simulink model "model_Q2"  (R2023b)
settings: Solver=ode45  StartTime=0.0  StopTime=25  RelTol=1e-5  AbsTol=1e-5  EnableMultiTasking=on
undefined symbols (not defined in the file or in its folder): control_Q2, vr
settings Model: Creator=pmorin  LastModifiedBy=baovi
settings SolverCC: AutoScaleAbsTol=off  AlgebraicLoopSolver=TrustRegion
settings DataIOCC: LimitDataPoints=on  SaveFormat=Array  SignalLoggingSaveFormat=ModelDataLogs  ReturnWorkspaceOutputs=off
settings OptimizationCC: BooleanDataType=off  ExpressionDepthLimit=2147483647  LifeSpan=inf
settings DebuggingCC: SaveWithParameterizedLinksMsg=none  UnderspecifiedInitializationDetection=Classic  MergeDetectMultiDrivingBlocksExec=none  SignalResolutionControl=TryResolveAllWithWarning  MultiTaskDSMMsg=warning  MultiTaskCondExecSysMsg=none  FcnCallInpInsideContextMsg=warning  UnconnectedInputMsg=warning  UnconnectedOutputMsg=warning  UnconnectedLineMsg=warning  StateNameClashWarn=warning  SFUnexpectedBacktrackingDiag=warning  SFNoUnconditionalDefaultTransitionDiag=warning  SFExecutionAtInitializationDiag=none  ArithmeticOperatorsInVariantConditions=warning
settings HardwareCC: ProdBitPerPointer=32  ProdBitPerSizeT=32  ProdBitPerPtrDiffT=32  ProdLargestAtomicFloat=None  ProdIntDivRoundTo=Undefined  ProdEndianess=Unspecified  ProdWordSize=32  ProdHWDeviceType=32-bit Generic  TargetUnknown=on
settings ModelReferenceCC: EnableRefExpFcnMdlSchedulingChecks=on  PropagateSignalLabelsOutOfModel=off
settings SFSimCC: SimUseLocalCustomCode=off  CustomCodeUndefinedFunction=UseInterfaceOnly
settings RTWCC: RTWUseLocalCustomCode=off
settings CodeAppCC: StateflowObjectComments=on
settings GRTTargetCC: TargetLangStandard=C89/C90 (ANSI)  CombineOutputUpdateFcns=off  GRTInterface=on
settings ConfigComp: CovMetricSettings=dw  CovSaveCumulativeToWorkspaceVar=on  CovSaveSingleToWorkspaceVar=on  CovExternalEMLEnable=off

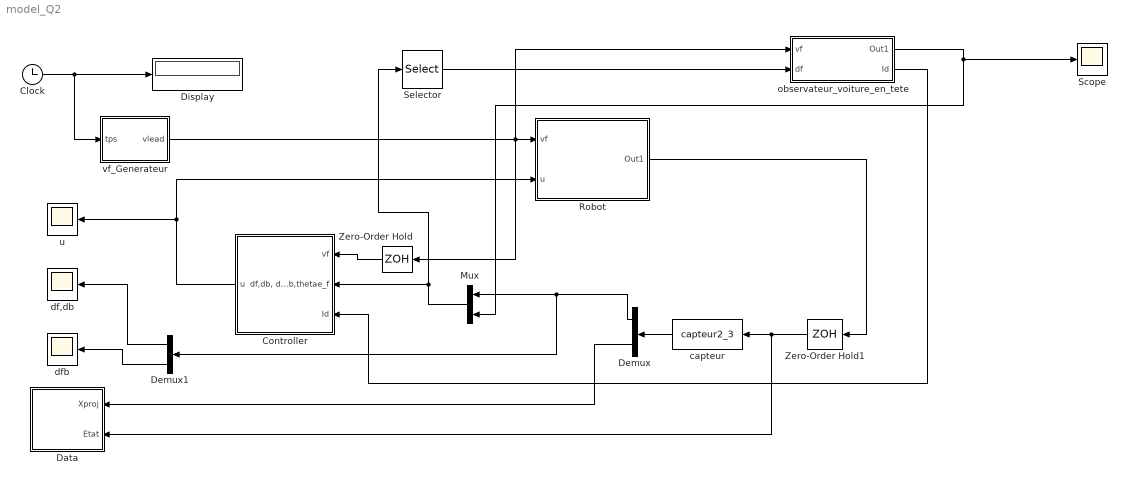
== system model_Q2 ==
  Clock : Clock
  Controller : Subsystem  mask{stomat=-1}
      mask prompts: stomat "Sample to matfile"
  Data : Subsystem  mask{stomat=-1}
      mask prompts: stomat "Sample to matfile"
  Demux : Demux  Outputs=[3;4]
  Demux1 : Demux  Outputs=[2;1]
  Display : Display
  Mux : Mux  Inputs=2
  Robot : Subsystem  mask{init=[5;10;0;2;4;-0.2]}
      mask prompts: init "Initial values"
  Scope : Scope
  Selector : Selector  InputPortWidth=5  IndexOptions=Index vector (dialog)  Indices=[1 ]  OutputSizes=1
  Zero-Order Hold : ZeroOrderHold  SampleTime=0.01
  Zero-Order Hold1 : ZeroOrderHold  SampleTime=0.01
  capteur : MATLABFcn  MATLABFcn=capteur2_3  OutputDimensions=7
  df,db : Scope
  dfb : Scope
  observateur_voiture_en_tete : Subsystem
  u : Scope
  vf_Generateur : Subsystem  mask{choix_traj=vitesse positive}
      mask prompts: choix_traj "trajectoire de reference"
      mask TypeOptions choix_traj: vitesse positive | vitesse quelconque
  wires:
  Clock/1 -> vf_Generateur/1(tps), Display/1
  Controller/1(u) -> Robot/2(u), u/1
  vf_Generateur/1("vlead ") -> Zero-Order Hold/1, observateur_voiture_en_tete/1(vf), Robot/1(vf)
  Robot/1(Out1) -> Zero-Order Hold1/1
  Zero-Order Hold/1 -> Controller/1(vf)
  Zero-Order Hold1/1 -> Data/2(Etat), capteur/1
  capteur/1 -> Demux/1
  Demux/2 -> Data/1(Xproj)
  Demux1/1 -> df,db/1
  Demux1/2 -> dfb/1
  Selector/1 -> observateur_voiture_en_tete/2(df)
  observateur_voiture_en_tete/1(Out1) -> Mux/2, Scope/1
  Demux/1 -> Demux1/1, Mux/1
  Mux/1 -> Controller/2("df,db, dfb,thetae_f"), Selector/1
  observateur_voiture_en_tete/2(Id) -> Controller/3(Id)

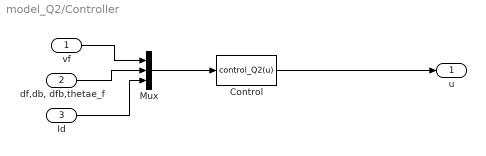
== system model_Q2/Controller ==
  vf : Inport
  "df,db, dfb,thetae_f" : Inport  Port=2
  Id : Inport  Port=3
  Control : MATLABFcn  MATLABFcn=control_Q2(u)  OutputDimensions=3
  Mux : Mux  Inputs=3
  u : Outport  VectorParamsAs1DForOutWhenUnconnected=off
  wires:
  Control/1 -> u/1
  vf/1 -> Mux/1
  "df,db, dfb,thetae_f"/1 -> Mux/2
  Mux/1 -> Control/1
  Id/1 -> Mux/3

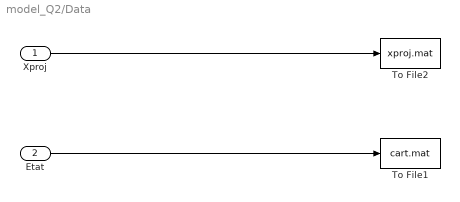
== system model_Q2/Data ==
  Xproj : Inport
  Etat : Inport  Port=2
  To File1 : ToFile  Filename=cart.mat  SampleTime=stomat
  To File2 : ToFile  Filename=xproj.mat  SampleTime=stomat
  wires:
  Etat/1 -> To File1/1
  Xproj/1 -> To File2/1

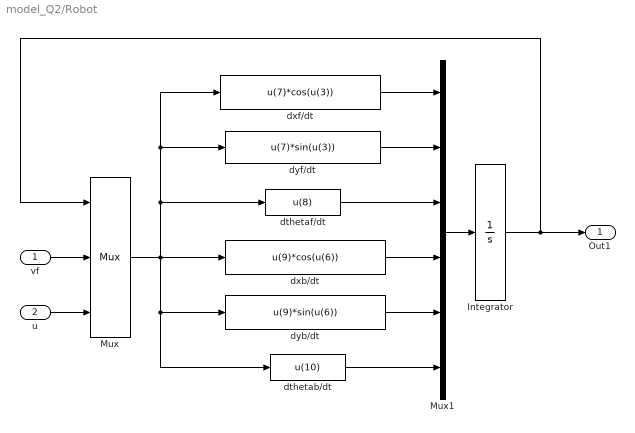
== system model_Q2/Robot ==
  vf : Inport
  u : Inport  Port=2
  Integrator : Integrator  InitialCondition=init
  Mux : Mux  Inputs=[6 1 3]
  Mux1 : Mux  Inputs=6
  dthetab/dt : Fcn  Expr=u(10)
  dthetaf/dt : Fcn  Expr=u(8)
  dxb/dt : Fcn  Expr=u(9)*cos(u(6))
  dxf/dt : Fcn  Expr=u(7)*cos(u(3))
  dyb/dt : Fcn  Expr=u(9)*sin(u(6))
  dyf/dt : Fcn  Expr=u(7)*sin(u(3))
  Out1 : Outport  VectorParamsAs1DForOutWhenUnconnected=off
  wires:
  vf/1 -> Mux/2
  Integrator/1 -> Out1/1, Mux/1
  Mux1/1 -> Integrator/1
  dxf/dt/1 -> Mux1/1
  dyf/dt/1 -> Mux1/2
  dthetaf/dt/1 -> Mux1/3
  u/1 -> Mux/3
  dxb/dt/1 -> Mux1/4
  dyb/dt/1 -> Mux1/5
  Mux/1 -> dxf/dt/1, dyf/dt/1, dthetaf/dt/1, dthetab/dt/1, dyb/dt/1, dxb/dt/1
  dthetab/dt/1 -> Mux1/6

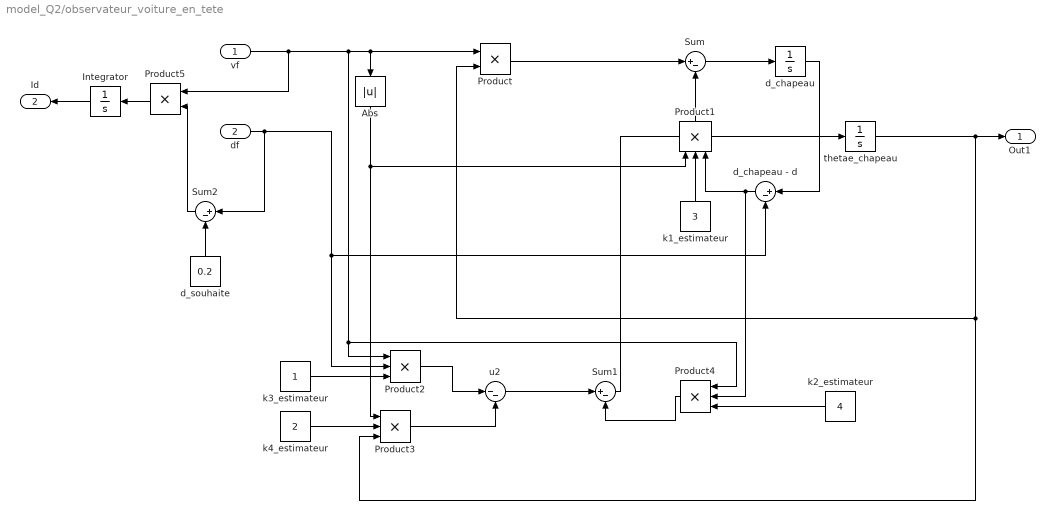
== system model_Q2/observateur_voiture_en_tete ==
  vf : Inport
  df : Inport  Port=2
  Abs : Abs  SaturateOnIntegerOverflow=off
  Integrator : Integrator
  Product : Product
  Product{1..4} (4 alike) : Product  Inputs=3
  Product5 : Product
  Sum : Sum  Inputs=|+-
  Sum1 : Sum  Inputs=|+-
  Sum2 : Sum  Inputs=|+-
  d_chapeau : Integrator
  d_chapeau - d : Sum  Inputs=|+-
  d_souhaite : Constant  Value=0.2
  k1_estimateur : Constant  Value=3
  k2_estimateur : Constant  Value=4
  k3_estimateur : Constant
  "k4_estimateur " : Constant  Value=2
  thetae_chapeau : Integrator
  u2 : Sum  Inputs=|--
  Out1 : Outport
  Id : Outport  Port=2
  wires:
  vf/1 -> Product5/1, Product4/1, Product2/1, Abs/1, Product/1
  thetae_chapeau/1 -> Product/2, Product3/3, Out1/1
  Product/1 -> Sum/1
  d_chapeau/1 -> d_chapeau - d/1
  df/1 -> Sum2/1, Product2/2, d_chapeau - d/2
  d_chapeau - d/1 -> Product1/3, Product4/2
  Product1/1 -> Sum/2
  Sum/1 -> d_chapeau/1
  Abs/1 -> Product3/1, Product1/1
  k1_estimateur/1 -> Product1/2
  k3_estimateur/1 -> Product2/3
  "k4_estimateur "/1 -> Product3/2
  Product2/1 -> u2/1
  Product3/1 -> u2/2
  u2/1 -> Sum1/1
  k2_estimateur/1 -> Product4/3
  Product4/1 -> Sum1/2
  Sum1/1 -> thetae_chapeau/1
  d_souhaite/1 -> Sum2/2
  Sum2/1 -> Product5/2
  Product5/1 -> Integrator/1
  Integrator/1 -> Id/1

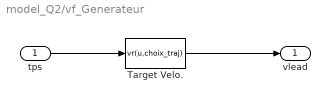
== system model_Q2/vf_Generateur ==
  tps : Inport
  Target Velo. : MATLABFcn  MATLABFcn=vr(u,choix_traj)  OutputDimensions=1
  "vlead " : Outport  VectorParamsAs1DForOutWhenUnconnected=off
  wires:
  Target Velo./1 -> "vlead "/1
  tps/1 -> Target Velo./1
